simulink model "Hana_Shamsaei_810600097_Rana_Heydari_810600071"  (R2022a)
settings: Solver=FixedStepAuto  StartTime=0.0  StopTime=50  FixedStep=0.01  RelTol=1e-3
undefined symbols (not defined in the file): C, F, K, m, M
settings Model: Creator=ansar  LastModifiedBy=Asus
settings ModelReferenceCC: EnableRefExpFcnMdlSchedulingChecks=off
settings RTWCC: Description=Generic Real-Time Target

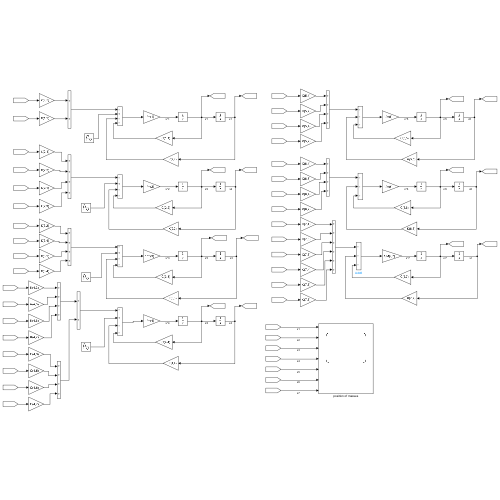
[thumbnail: Simulink's stored preview of the top-level diagram]
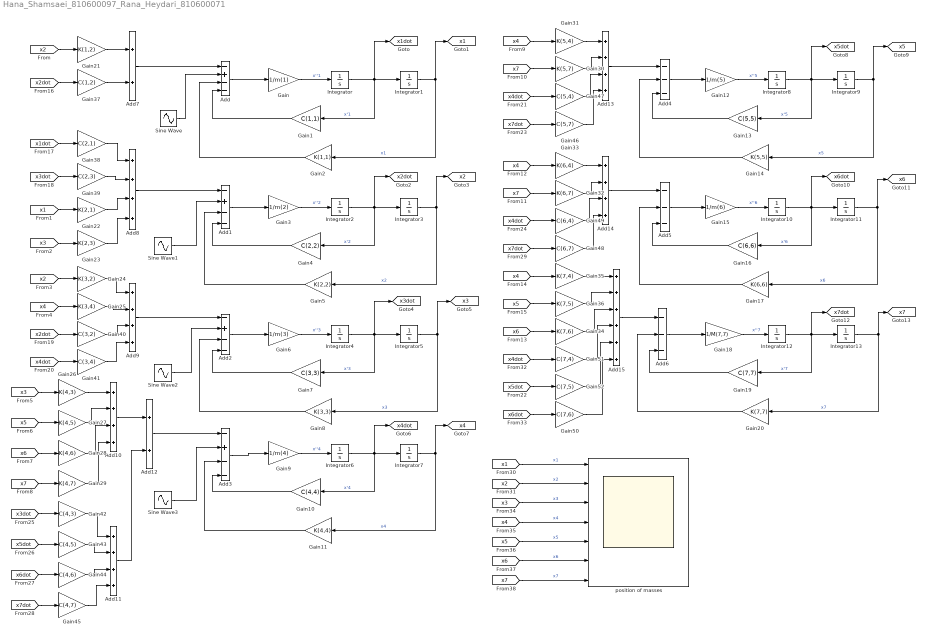
== system Hana_Shamsaei_810600097_Rana_Heydari_810600071 ==
  Add{,1..3} (4 alike) : Sum  Inputs=-+--
  Add{8..11,13..14} (6 alike) : Sum  Inputs=++++
  Add12 : Sum
  Add15 : Sum  Inputs=++++++
  Add4 : Sum  Inputs=---
  Add5 : Sum  Inputs=---
  Add6 : Sum  Inputs=---
  Add7 : Sum
  Gain : Gain  Gain=1/m(1)
  Gain1 : Gain  Gain=C(1,1)
  Gain10 : Gain  Gain=C(4,4)
  Gain11 : Gain  Gain=K(4,4)
  Gain12 : Gain  Gain=1/m(5)
  Gain13 : Gain  Gain=C(5,5)
  Gain14 : Gain  Gain=K(5,5)
  Gain15 : Gain  Gain=1/m(6)
  Gain16 : Gain  Gain=C(6,6)
  Gain17 : Gain  Gain=K(6,6)
  Gain18 : Gain  Gain=1/M(7,7)
  Gain19 : Gain  Gain=C(7,7)
  Gain2 : Gain  Gain=K(1,1)
  Gain20 : Gain  Gain=K(7,7)
  Gain21 : Gain  Gain=K(1,2)
  Gain22 : Gain  Gain=K(2,1)
  Gain23 : Gain  Gain=K(2,3)
  Gain24 : Gain  Gain=K(3,2)
  Gain25 : Gain  Gain=K(3,4)
  Gain26 : Gain  Gain=K(4,3)
  Gain27 : Gain  Gain=K(4,5)
  Gain28 : Gain  Gain=K(4,6)
  Gain29 : Gain  Gain=K(4,7)
  Gain3 : Gain  Gain=1/m(2)
  Gain30 : Gain  Gain=K(5,7)
  Gain31 : Gain  Gain=K(5,4)
  Gain32 : Gain  Gain=K(6,7)
  Gain33 : Gain  Gain=K(6,4)
  Gain34 : Gain  Gain=K(7,6)
  Gain35 : Gain  Gain=K(7,4)
  Gain36 : Gain  Gain=K(7,5)
  Gain37 : Gain  Gain=C(1,2)
  Gain38 : Gain  Gain=C(2,1)
  Gain39 : Gain  Gain=C(2,3)
  Gain4 : Gain  Gain=C(2,2)
  Gain40 : Gain  Gain=C(3,2)
  Gain41 : Gain  Gain=C(3,4)
  Gain42 : Gain  Gain=C(4,3)
  Gain43 : Gain  Gain=C(4,5)
  Gain44 : Gain  Gain=C(4,6)
  Gain45 : Gain  Gain=C(4,7)
  Gain46 : Gain  Gain=C(5,7)
  Gain47 : Gain  Gain=C(5,4)
  Gain48 : Gain  Gain=C(6,7)
  Gain49 : Gain  Gain=C(6,4)
  Gain5 : Gain  Gain=K(2,2)
  Gain50 : Gain  Gain=C(7,6)
  Gain51 : Gain  Gain=C(7,4)
  Gain52 : Gain  Gain=C(7,5)
  Gain6 : Gain  Gain=1/m(3)
  Gain7 : Gain  Gain=C(3,3)
  Gain8 : Gain  Gain=K(3,3)
  Gain9 : Gain  Gain=1/m(4)
  Integrator{,1..12} (13 alike) : Integrator
  Integrator13 : Integrator  InitialCondition=-8*pi/180
  Sine Wave : Sin  Amplitude=F(1)  Frequency=1.75  SampleTime=0
  Sine Wave1 : Sin  Amplitude=F(2)  Frequency=1.75  SampleTime=0
  Sine Wave2 : Sin  Amplitude=F(3)  Frequency=1.75  SampleTime=0
  Sine Wave3 : Sin  Amplitude=F(4)  Frequency=1.75  SampleTime=0
  position of masses : Scope  NumInputPorts=7
  tag scope: x1=global, x1dot=global, x2=global, x2dot=global, x3=global, x3dot=global, x4=global, x4dot=global, x5=global, x5dot=global, x6=global, x6dot=global, x7=global, x7dot=global
  wires:
  Add/1 -> Gain/1
  Gain/1 -> Integrator/1  "x''1"
  Integrator/1 -> Integrator1/1, [x1dot], Gain1/1  "x'1"
  Integrator1/1 -> [x1], Gain2/1  "x1"
  Integrator2/1 -> Gain4/1, [x2dot], Integrator3/1  "x'2"
  Add1/1 -> Gain3/1
  Gain3/1 -> Integrator2/1  "x''2"
  Integrator3/1 -> Gain5/1, [x2]  "x2"
  Integrator5/1 -> Gain8/1, [x3]  "x3"
  Gain6/1 -> Integrator4/1  "x''3"
  Add2/1 -> Gain6/1
  Integrator4/1 -> Gain7/1, [x3dot], Integrator5/1  "x'3"
  Add3/1 -> Gain9/1
  Gain9/1 -> Integrator6/1  "x''4"
  Integrator7/1 -> Gain11/1, [x4]  "x4"
  Integrator6/1 -> Gain10/1, [x4dot], Integrator7/1  "x'4"
  Gain14/1 -> Add4/2
  Add4/1 -> Gain12/1
  Gain13/1 -> Add4/3
  Gain12/1 -> Integrator8/1  "x''5"
  Integrator9/1 -> [x5], Gain14/1  "x5"
  Integrator8/1 -> Gain13/1, [x5dot], Integrator9/1  "x'5"
  Gain17/1 -> Add5/2
  Add5/1 -> Gain15/1
  Gain16/1 -> Add5/3
  Gain15/1 -> Integrator10/1  "x''6"
  Integrator11/1 -> [x6], Gain17/1  "x6"
  Integrator10/1 -> Gain16/1, [x6dot], Integrator11/1  "x'6"
  Gain20/1 -> Add6/2
  Add6/1 -> Gain18/1
  Gain19/1 -> Add6/3
  Gain18/1 -> Integrator12/1  "x''7"
  Integrator13/1 -> Gain20/1, [x7]  "x7"
  Integrator12/1 -> Gain19/1, [x7dot], Integrator13/1  "x'7"
  [x4] -> Gain31/1
  [x7] -> Gain30/1
  [x7] -> Gain32/1
  [x4] -> Gain33/1
  [x4] -> Gain35/1
  [x6] -> Gain34/1
  [x5] -> Gain36/1
  [x2] -> Gain21/1
  Gain21/1 -> Add7/1
  Gain37/1 -> Add7/2
  [x2dot] -> Gain37/1
  [x3] -> Gain23/1
  [x1] -> Gain22/1
  [x1dot] -> Gain38/1
  [x3dot] -> Gain39/1
  Gain38/1 -> Add8/1
  Gain39/1 -> Add8/2
  Gain22/1 -> Add8/3
  Gain23/1 -> Add8/4
  [x2] -> Gain24/1
  [x4] -> Gain25/1
  Gain25/1 -> Add9/2
  Gain24/1 -> Add9/1
  [x4dot] -> Gain41/1
  [x2dot] -> Gain40/1
  Gain40/1 -> Add9/3
  Gain41/1 -> Add9/4
  [x5] -> Gain27/1
  [x3] -> Gain26/1
  [x6] -> Gain28/1
  Gain26/1 -> Add10/1
  Gain27/1 -> Add10/2
  Gain28/1 -> Add10/3
  Gain29/1 -> Add10/4
  Gain42/1 -> Add11/1
  [x6dot] -> Gain44/1
  [x7dot] -> Gain45/1
  Gain44/1 -> Add11/3
  [x3dot] -> Gain42/1
  [x5dot] -> Gain43/1
  Gain45/1 -> Add11/4
  Gain43/1 -> Add11/2
  Add10/1 -> Add12/1
  Add11/1 -> Add12/2
  [x4dot] -> Gain47/1
  [x7dot] -> Gain46/1
  Gain47/1 -> Add13/3
  Gain30/1 -> Add13/2
  Gain31/1 -> Add13/1
  Gain46/1 -> Add13/4
  [x7dot] -> Gain48/1
  [x4dot] -> Gain49/1
  Gain33/1 -> Add14/1
  Gain32/1 -> Add14/2
  Gain49/1 -> Add14/3
  Gain48/1 -> Add14/4
  Add14/1 -> Add5/1
  [x5dot] -> Gain52/1
  [x6dot] -> Gain50/1
  [x4dot] -> Gain51/1
  Gain35/1 -> Add15/1
  Gain36/1 -> Add15/2
  Gain34/1 -> Add15/3
  Gain51/1 -> Add15/4
  Gain52/1 -> Add15/5
  Gain50/1 -> Add15/6
  Add15/1 -> Add6/1
  [x1] -> position of masses/1  "x1"
  [x2] -> position of masses/2  "x2"
  [x3] -> position of masses/3  "x3"
  [x4] -> position of masses/4  "x4"
  [x5] -> position of masses/5  "x5"
  [x6] -> position of masses/6  "x6"
  [x7] -> position of masses/7  "x7"
  Gain1/1 -> Add/4
  Gain2/1 -> Add/3
  Sine Wave/1 -> Add/2
  Add7/1 -> Add/1
  Sine Wave1/1 -> Add1/2
  Gain4/1 -> Add1/4
  Gain5/1 -> Add1/3
  Add8/1 -> Add1/1
  Gain7/1 -> Add2/4
  Gain8/1 -> Add2/3
  Sine Wave2/1 -> Add2/2
  Add9/1 -> Add2/1
  Sine Wave3/1 -> Add3/2
  Gain10/1 -> Add3/4
  Gain11/1 -> Add3/3
  Add12/1 -> Add3/1
  [x7] -> Gain29/1
  Add13/1 -> Add4/1
